simulink model "deney41"  (R2023b)
settings: Solver=VariableStepAuto  StartTime=0.0  StopTime=50  RelTol=1e-3
libraries: commrandsrc3 x1, dspfdesign x1
settings Model: Creator=fatih  LastModifiedBy=fatih

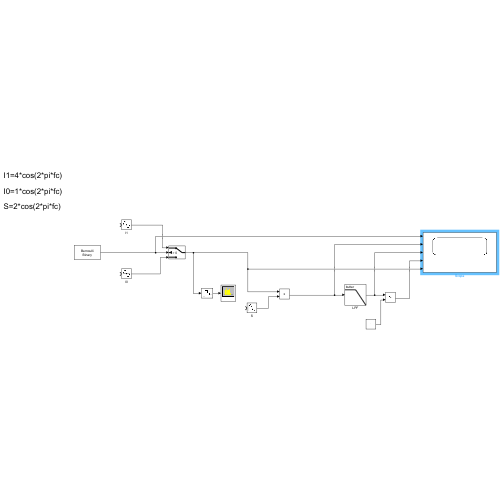
[thumbnail: Simulink's stored preview of the top-level diagram]
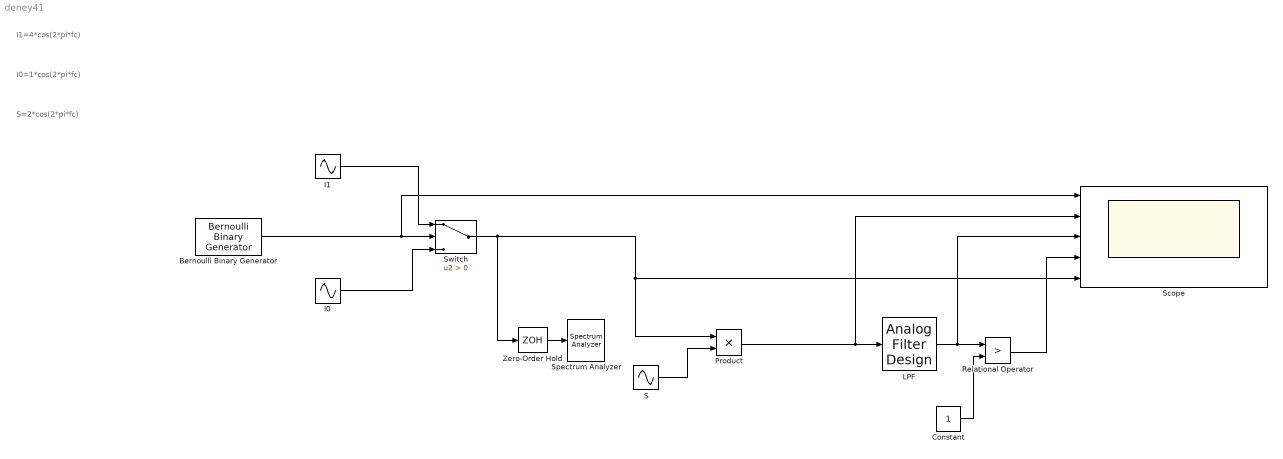
== system deney41 ==
  note: S=2*cos(2*pi*fc)
  note: I0=1*cos(2*pi*fc)
  note: I1=4*cos(2*pi*fc)
  Bernoulli Binary Generator : commrandsrc3/Bernoulli Binary Generator  ProbabilityOfZero=0.5  SeedSource=Auto  Seed=0  SampleTime=1  SamplesPerFrame=1  OutputDataType=double  SimulateUsing=Interpreted execution
  Constant : Constant
  I0 : Sin  TimeSource=Use external signal  Frequency=12.56663706  Phase=pi/2  SampleTime=0
  I1 : Sin  TimeSource=Use external signal  Amplitude=4  Frequency=12.5663706  Phase=pi/2  SampleTime=0
  LPF : dspfdesign/Analog Filter Design  method=Butterworth  filttype=Lowpass  N=8  Wlo=1.5*2*pi  Whi=80  Rp=2  Rs=40
  Product : Product
  Relational Operator : RelationalOperator  Operator=>  OutDataTypeStr=boolean  RndMeth=Simplest  InputSameDT=off
  S : Sin  TimeSource=Use external signal  Amplitude=2  Frequency=12.5663706  Phase=pi  SampleTime=0
  Scope : Scope  NumInputPorts=5
  Spectrum Analyzer : SpectrumAnalyzer  WindowPosition=[1.000000,41.000000,1366.000000,705.000000,]  ScopeFrameLocation=window  Span=100  StartFrequency=-50  StopFrequency=50  YLimits=[-96.01455601,-5.66483422]  ShowLegend=on  ExpandToolstrip=on
      settings: OpenAtSimulationStart=off
  Switch : Switch  Criteria=u2 > Threshold  SaturateOnIntegerOverflow=off  InputSameDT=off
  Zero-Order Hold : ZeroOrderHold  SampleTime=0.01
  wires:
  Switch/1 -> Product/1, Scope/5, Zero-Order Hold/1
  Zero-Order Hold/1 -> Spectrum Analyzer/1
  I1/1 -> Switch/1
  I0/1 -> Switch/3
  S/1 -> Product/2
  Constant/1 -> Relational Operator/2
  Bernoulli Binary Generator/1 -> Scope/1, Switch/2
  Product/1 -> LPF/1, Scope/2
  Relational Operator/1 -> Scope/4
  LPF/1 -> Scope/3, Relational Operator/1
